simulink model "prototipo"  (R2022b)
settings: Solver=ode3  StartTime=0.0  StopTime=10  RelTol=1e-3  EnableMultiTasking=on
model workspace (MAT data in the model file):
  RGBData = [62 63 65 64 60 62 65 62 60 59 59 59 ... (230400 elements, 320x240x3)]
libraries: sensehatlib x2, raspberrypiAVlib x2, visionanalysis x1, visiontextngfix x1
(part 2 of 2)

== matlab function prototipo/MATLAB Function1 ==
  data: i input; r output size=[224 224]; g output size=[224 224]; b output size=[224 224]
function [r,g,b] = ImageToRGB(i)
%#codegen
r =i(:,:,1);
g =i(:,:,2);
b =i(:,:,3);
end

== matlab function prototipo/MATLAB Function ==
  data: image input; output output; label input

function output = addLabel(image,label)
%#codegen
label_str = cellstr(label);
text2display = sprintf("Label : %s \nScore: %f", label_str{:}, max_score);
% Para la generación de código, text2display necesita ser de tipo cell
% en vez de string
%ctext2display = cellstr(text2display);
% Insertamos en img, en la posición 0,0, el texto previamente calculado
output = insertText(image, [0,0], text2display);
end

== matlab function prototipo/MATLAB Function4 ==
  data: img input; bounding_boxes output size=[424 424]; img_resized output size=[224 224 3]
function [bounding_boxes,img_resized] = detectorYOLO(img)

input_size = [224,224,3];

detector = coder.loadDeepLearningNetwork("C:\Users\alber\My Documents\Universidad\4\TFG\Smart Hive\SAVED_OBJECTS\YOLOTY\2\detector.mat");
bounding_boxes = detect(detector,img);

% Si no es vacío, es decir, ha detectado alguna cara.
if ~isempty(bounding_boxes)
    % La recortamos para solo quedarnos con la cara detectado.
    img_processed = imcrop(img, bounding_boxes(1,:));
    % Para que cuando lo implemento en la Rasp, sepa que la matriz
    % tiene "dimensión 3" en la tercera dimensión.
    img_processed = img_processed(:,:, 1:3);

    % Adaptamos el tamaño de la imagen a la entrada de la red.
    img_resized = imresize(img_processed, input_size(1:2));
end
end

== matlab function prototipo/MATLAB Function3 ==
  data: bounding_boxes input; img_resized input; img_label output size=[224 224 3]
function img_label = classification(bounding_boxes,img_resized)

net = coder.loadDeepLearningNetwork("./SAVED_OBJECTS/net.mat");

% Clasificamos la imagen
[label,score] = net.classify(img_resized);
max_score = max(score);

%label_str = cellstr(label);
text2display = sprintf("Label : %s \nScore: %f", label, max_score);

img_label = insertText(img, [0,0], text2display);
% Actualizamos el cuadrado solamente si ha detectado una cara.
if ~isempty(bounding_boxes)
    img_label = insertObjectAnnotation(img_label, "rectangle", bounding_boxes, label, "LineWidth", 2);
end
end
